simulink model "pendule_inv_etu1"  (R2021a)
settings: Solver=VariableStepAuto  StartTime=0.0  StopTime=10.0  RelTol=1e-3
values from neighbouring files (symbols this model uses):
  g = 9.81    [simu_pendule_inv_capteur_etu.m]    (also in simu_pendule_inv_echant_etu.m; simu_pendule_inv_etu.m)
  K = [10 1]    [simu_pendule_inv_capteur_etu.m]    (also in simu_pendule_inv_echant_etu.m = [30 10]; simu_pendule_inv_etu.m = [30 10])
  l = 10    [simu_pendule_inv_capteur_etu.m]    (also in simu_pendule_inv_echant_etu.m; simu_pendule_inv_etu.m)
  ue = 0    [simu_pendule_inv_capteur_etu.m]    (also in simu_pendule_inv_echant_etu.m; simu_pendule_inv_etu.m)
  x0 = [pi/20 0]'    [simu_pendule_inv_capteur_etu.m]    (also in simu_pendule_inv_echant_etu.m; simu_pendule_inv_etu.m = [pi/10 0]')
  xe = [0 0]'    [simu_pendule_inv_capteur_etu.m]    (also in simu_pendule_inv_echant_etu.m; simu_pendule_inv_etu.m)
settings Model: Creator=maimi  LastModifiedBy=Jed

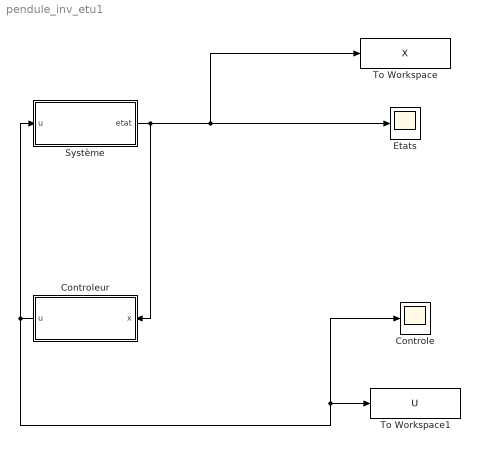
== system pendule_inv_etu1 ==
  Controle : Scope
  Controleur : Subsystem
  Etats : Scope
  Système : Subsystem
  To Workspace : ToWorkspace  VariableName=X  SaveFormat=Timeseries  SampleTime=-1
  To Workspace1 : ToWorkspace  VariableName=U  SaveFormat=Timeseries  SampleTime=-1
      settings: Save2DSignal=2-D array (concatenate along first dimension)
  wires:
  Controleur/1(u) -> Système/1(u), To Workspace1/1, Controle/1
  Système/1(etat) -> Controleur/1(x), To Workspace/1, Etats/1

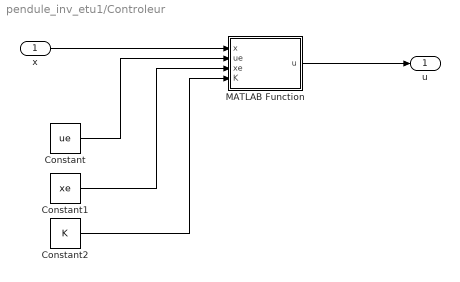
== system pendule_inv_etu1/Controleur ==
  x : Inport
  Constant : Constant  Value=ue
  Constant1 : Constant  Value=xe
  Constant2 : Constant  Value=K
  MATLAB Function : MATLAB Function  TreatAsAtomicUnit=on
  u : Outport
  wires:
  MATLAB Function/1(u) -> u/1
  Constant/1 -> MATLAB Function/2(ue)
  Constant1/1 -> MATLAB Function/3(xe)
  Constant2/1 -> MATLAB Function/4(K)
  x/1 -> MATLAB Function/1(x)

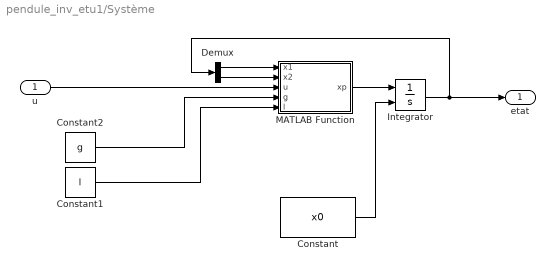
== system pendule_inv_etu1/Système ==
  u : Inport
  Constant : Constant  Value=x0
  Constant1 : Constant  Value=l
  Constant2 : Constant  Value=g
  Demux : Demux  Outputs=2
  Integrator : Integrator  InitialConditionSource=external
  MATLAB Function : MATLAB Function  TreatAsAtomicUnit=on
  etat : Outport
  wires:
  Integrator/1 -> etat/1, Demux/1
  Demux/1 -> MATLAB Function/1(x1)
  Demux/2 -> MATLAB Function/2(x2)
  MATLAB Function/1(xp) -> Integrator/1
  Constant/1 -> Integrator/2
  u/1 -> MATLAB Function/3(u)
  Constant2/1 -> MATLAB Function/4(g)
  Constant1/1 -> MATLAB Function/5(l)

== matlab function pendule_inv_etu1/Controleur/MATLAB Function ==
  data: x input size=[2 1]; u output size=1; ue input size=1; xe input size=[2 1]; K input size=[1 2]
function u = fcn(x, ue, xe, K)

u = ue + K*(x - xe);

== matlab function pendule_inv_etu1/Système/MATLAB Function ==
  data: x1 input size=1; x2 input size=1; u input size=1; xp output size=[2 1]; g input size=1; l input size=1
function xp = fcn(x1, x2, u, g, l)
x1p = x2;
x2p = g/l*sin(x1) - (cos(x1)*u)/l;
xp = [x1p; x2p];
